simulink model "Termin2VE"  (Simulink 8.3)
settings: Solver=ode3  StartTime=0.0  StopTime=512/8000  FixedStep=1/8000  RelTol=1e-3
undefined symbols (not defined in the file or in its folder): get
libraries: dspsnks4 x4, dspxfrm3 x2, dspsrcs4 x2, dspsigops x2
settings Model: Creator=dsv1_5  LastModifiedBy=dsv1_5
settings DataIOCC: SignalLoggingSaveFormat=Dataset
settings DebuggingCC: UnderspecifiedInitializationDetection=Simplified  StateNameClashWarn=none
settings GRTTargetCC: CombineOutputUpdateFcns=on  GRTInterface=off

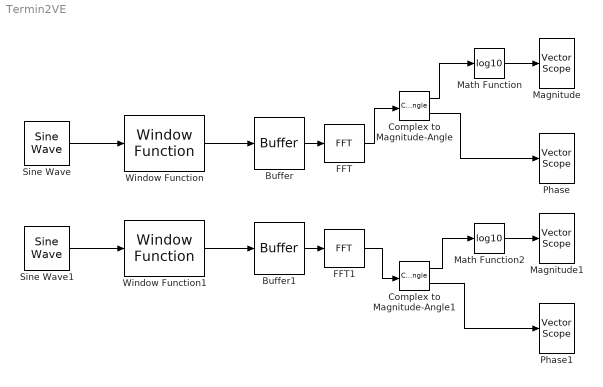
== system Termin2VE ==
  Buffer : Buffer  N=512  TreatMby1Signals=One channel
  Buffer1 : Buffer  N=512  TreatMby1Signals=One channel
  Complex to Magnitude-Angle : ComplexToMagnitudeAngle
  Complex to Magnitude-Angle1 : ComplexToMagnitudeAngle
  FFT : dspxfrm3/FFT  CompMethod=Table lookup  TableOpt=NEW  TableOptActive=Speed  BitRevOrder=off  InheritFFTLength=on  FFTLength=64  WrapInput=on  RowConvenienceOn=on  FFTImplementation=Auto  SkipNorm=off  firstCoeffDataTypeStr=Inherit: Same word length as input  firstCoeffLastDataTypeStr=Inherit: Same word length as input  outputMin=[]  outputMax=[]  roundingMode=Floor  overflowMode=off
  FFT1 : dspxfrm3/FFT  CompMethod=Table lookup  TableOpt=NEW  TableOptActive=Speed  BitRevOrder=off  InheritFFTLength=on  FFTLength=64  WrapInput=on  RowConvenienceOn=on  FFTImplementation=Auto  SkipNorm=off  firstCoeffDataTypeStr=Inherit: Same word length as input  firstCoeffLastDataTypeStr=Inherit: Same word length as input  outputMin=[]  outputMax=[]  roundingMode=Floor  overflowMode=off
  Magnitude : dspsnks4/Vector Scope  ScopeProperties=on  Domain=Time  HorizSpan=1  DisplayProperties=off  AxisGrid=on  Memory=off  FrameNumber=on  AxisLegend=off  AxisZoom=off  OpenScopeAtSimStart=on  OpenScopeImmediately=off  FigPos=get(0,'defaultfigureposition')  AxisProperties=off  XUnits=Hertz  XRange=[0...Fs/2]  InheritXIncr=on  XIncr=1  XLabel=Time  XLimit=Auto  XMin=0  XMax=1  XStart=0  YUnits=dB  YLabel=Amplitude  LineProperties=off  XAxisParamsVer=6.9
      settings: YMin=-10  YMax=10
  Magnitude1 : dspsnks4/Vector Scope  ScopeProperties=on  Domain=Time  HorizSpan=1  DisplayProperties=off  AxisGrid=on  Memory=off  FrameNumber=on  AxisLegend=off  AxisZoom=off  OpenScopeAtSimStart=on  OpenScopeImmediately=off  FigPos=get(0,'defaultfigureposition')  AxisProperties=off  XUnits=Hertz  XRange=[0...Fs/2]  InheritXIncr=on  XIncr=1  XLabel=Time  XLimit=Auto  XMin=0  XMax=1  XStart=0  YUnits=dB  YLabel=Amplitude  LineProperties=off  XAxisParamsVer=6.9
      settings: YMin=-10  YMax=10
  Math Function : Math  Operator=log10  SaturateOnIntegerOverflow=on
  Math Function2 : Math  Operator=log10  SaturateOnIntegerOverflow=on
  Phase : dspsnks4/Vector Scope  ScopeProperties=on  Domain=Time  HorizSpan=1  DisplayProperties=off  AxisGrid=on  Memory=off  FrameNumber=on  AxisLegend=off  AxisZoom=off  OpenScopeAtSimStart=on  OpenScopeImmediately=off  FigPos=get(0,'defaultfigureposition')  AxisProperties=off  XUnits=Hertz  XRange=[0...Fs/2]  InheritXIncr=on  XIncr=1  XLabel=Time  XLimit=Auto  XMin=0  XMax=1  XStart=0  YUnits=dB  YLabel=Amplitude  LineProperties=off  XAxisParamsVer=6.9
      settings: YMin=-10  YMax=10
  Phase1 : dspsnks4/Vector Scope  ScopeProperties=on  Domain=Time  HorizSpan=1  DisplayProperties=off  AxisGrid=on  Memory=off  FrameNumber=on  AxisLegend=off  AxisZoom=off  OpenScopeAtSimStart=on  OpenScopeImmediately=off  FigPos=get(0,'defaultfigureposition')  AxisProperties=off  XUnits=Hertz  XRange=[0...Fs/2]  InheritXIncr=on  XIncr=1  XLabel=Time  XLimit=Auto  XMin=0  XMax=1  XStart=0  YUnits=dB  YLabel=Amplitude  LineProperties=off  XAxisParamsVer=6.9
      settings: YMin=-10  YMax=10
  Sine Wave : dspsrcs4/Sine Wave  Amplitude=1  Frequency=500  Phase=0  SampleMode=Discrete  OutComplex=Real  CompMethod=Trigonometric fcn  TableSize=Speed  SampleTime=1/8000  SamplesPerFrame=1  ResetState=Restart at time zero  dataType=double  wordLen=16  udDataType=sfix(16)  fracBitsMode=Best precision  numFracBits=15  OutDataTypeStr=double  LastOutDataTypeStr=double
  Sine Wave1 : dspsrcs4/Sine Wave  Amplitude=1  Frequency=510  Phase=0  SampleMode=Discrete  OutComplex=Real  CompMethod=Trigonometric fcn  TableSize=Speed  SampleTime=1/8000  SamplesPerFrame=1  ResetState=Restart at time zero  dataType=double  wordLen=16  udDataType=sfix(16)  fracBitsMode=Best precision  numFracBits=15  OutDataTypeStr=double  LastOutDataTypeStr=double
  Window Function : dspsigops/Window Function  winmode=Apply window to input  wintype=Boxcar  sampmode=Continuous  samptime=1  N=64  Rs=50  beta=10  winsamp=Symmetric  UserWindow=hamming  OptParams=off  UserParams={'symmetric'}  RowConvenienceOn=on  dataType=double  isSigned=on  wordLen=16  udDataType=sfix(16)  fracBitsMode=Best precision  numFracBits=15  roundingMode=Floor  overflowMode=off  numSidelobes=4  sidelobeLevel=-30
  Window Function1 : dspsigops/Window Function  winmode=Apply window to input  wintype=Hanning  sampmode=Continuous  samptime=1  N=64  Rs=50  beta=10  winsamp=Symmetric  UserWindow=hamming  OptParams=off  UserParams={'symmetric'}  RowConvenienceOn=on  dataType=double  isSigned=on  wordLen=16  udDataType=sfix(16)  fracBitsMode=Best precision  numFracBits=15  roundingMode=Floor  overflowMode=off  numSidelobes=4  sidelobeLevel=-30
  wires:
  Window Function/1 -> Buffer/1
  Buffer/1 -> FFT/1
  FFT/1 -> Complex to Magnitude-Angle/1
  Complex to Magnitude-Angle/1 -> Math Function/1
  Sine Wave/1 -> Window Function/1
  Window Function1/1 -> Buffer1/1
  Buffer1/1 -> FFT1/1
  FFT1/1 -> Complex to Magnitude-Angle1/1
  Complex to Magnitude-Angle1/1 -> Math Function2/1
  Math Function/1 -> Magnitude/1
  Complex to Magnitude-Angle/2 -> Phase/1
  Math Function2/1 -> Magnitude1/1
  Complex to Magnitude-Angle1/2 -> Phase1/1
  Sine Wave1/1 -> Window Function1/1
